simulink model "SimulinkModelGeneral_Cascaded_BAv03"  (R2022b)
settings: Solver=VariableStepAuto  StartTime=0.0  StopTime=9*3600  MaxStep=0.2  RelTol=1e-3
settings Model: NumberOfSteps=100  Creator=giaco  LastModifiedBy=giaco

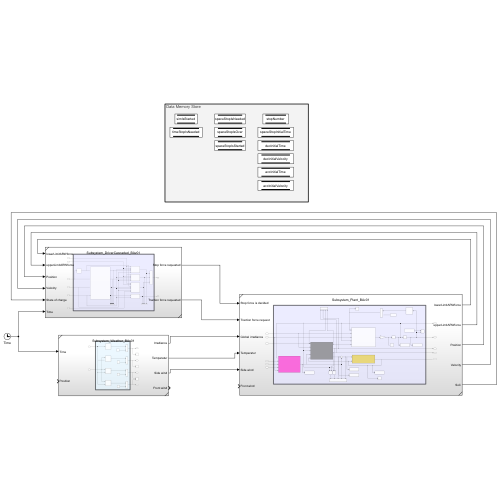
[thumbnail: Simulink's stored preview of the top-level diagram]
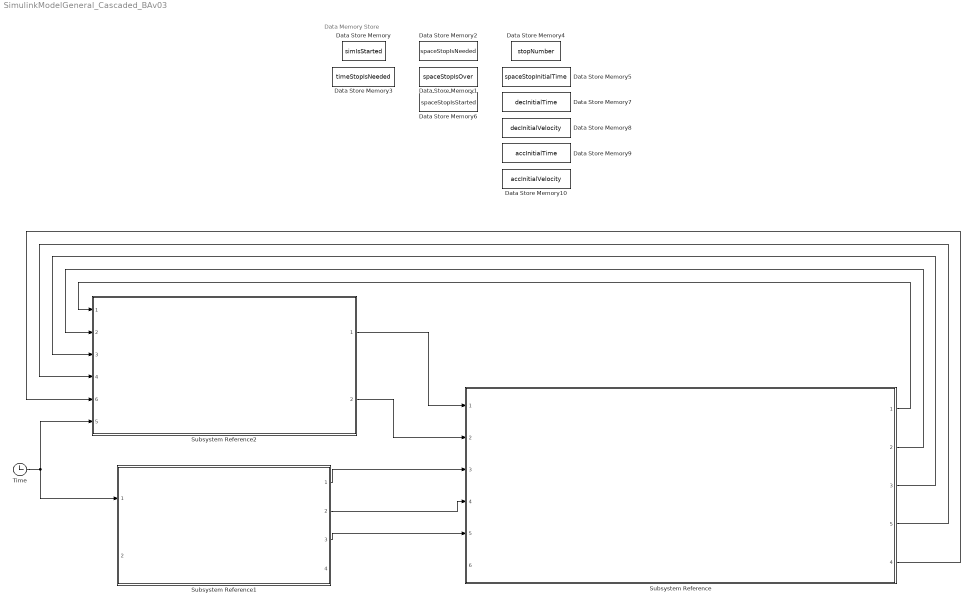
== system SimulinkModelGeneral_Cascaded_BAv03 ==
  note: Data Memory Store
  Data Store Memory : DataStoreMemory  DataStoreName=simIsStarted  WriteAfterWriteMsg=warning  InitialValue=true  ShowAdditionalParam=off  OutDataTypeStr=boolean
  Data Store Memory1 : DataStoreMemory  DataStoreName=spaceStopIsOver  WriteAfterWriteMsg=warning  InitialValue=false  ShowAdditionalParam=off  OutDataTypeStr=boolean
  Data Store Memory10 : DataStoreMemory  DataStoreName=accInitialVelocity  WriteAfterWriteMsg=warning  VectorParams1D=off  ShowAdditionalParam=off  OutDataTypeStr=double
  Data Store Memory2 : DataStoreMemory  DataStoreName=spaceStopIsNeeded  WriteAfterWriteMsg=warning  InitialValue=false  ShowAdditionalParam=off  OutDataTypeStr=boolean
  Data Store Memory3 : DataStoreMemory  DataStoreName=timeStopIsNeeded  WriteAfterWriteMsg=warning  InitialValue=false  ShowAdditionalParam=off  OutDataTypeStr=boolean
  Data Store Memory4 : DataStoreMemory  DataStoreName=stopNumber  WriteAfterWriteMsg=warning  InitialValue=2  VectorParams1D=off  ShowAdditionalParam=off  OutDataTypeStr=int8
  Data Store Memory5 : DataStoreMemory  DataStoreName=spaceStopInitialTime  WriteAfterWriteMsg=warning  VectorParams1D=off  ShowAdditionalParam=off  OutDataTypeStr=double
  Data Store Memory6 : DataStoreMemory  DataStoreName=spaceStopIsStarted  WriteAfterWriteMsg=warning  InitialValue=false  ShowAdditionalParam=off  OutDataTypeStr=boolean
  Data Store Memory7 : DataStoreMemory  DataStoreName=decInitialTime  WriteAfterWriteMsg=warning  VectorParams1D=off  ShowAdditionalParam=off  OutDataTypeStr=double
  Data Store Memory8 : DataStoreMemory  DataStoreName=decInitialVelocity  WriteAfterWriteMsg=warning  VectorParams1D=off  ShowAdditionalParam=off  OutDataTypeStr=double
  Data Store Memory9 : DataStoreMemory  DataStoreName=accInitialTime  WriteAfterWriteMsg=warning  VectorParams1D=off  ShowAdditionalParam=off  OutDataTypeStr=double
  Subsystem Reference : Subsystem  ReferencedSubsystem=Subsystem_Plant_BAv01
      settings: PortSchema="{\"entries\":[{\"content\":{\"sides\":[{\"content\":{\"connectorIds\":[\"In1\",\"In2\",\"In3\",\"In4\",\"In5\",\"In6\"]},\"type\":\"ConnectorPlacement.EquallySpacedRectSide\",\"uuid\":\"201c7402-5e26-4969-bf95-741aace5d52f\"},{\"content\":{\"connectorIds\":[\"Out1\",\"Out2\",\"Out3\",\"Out5\",\"Out4\"],\"side\":\"RIGHT\"},\"type\":\"ConnectorPlacement.EquallySpacedRectSide\",\"uuid\":\"eac15500-2534-4791-a6c9-7cdce956e4c6\"},{\"content\":{\"connectorIds\":[],\"side\":\"TOP\"},\"type\":\"ConnectorPlacement.EquallySpacedRectSide\",\"uuid\":\"55480481-707b-452f-a9f7-06d47dfb860c\"}]},\"type\":\"ConnectorPlacement.EquallySpacedConnector\",\"uuid\":\"eb257ac9-5ab4-418c-93e8-134a72900e24\"}],\"packageUris\":[\"http://schema.mathworks.com/mf0/Connector/R2020b\"],\"version\":\"1.0\"}"
  Subsystem Reference1 : Subsystem  ReferencedSubsystem=Subsystem_Weather_BAv01
  Subsystem Reference2 : Subsystem  ReferencedSubsystem=Subsystem_DriverCascaded_BAv01
      settings: PortSchema="{\"entries\":[{\"content\":{\"sides\":[{\"content\":{\"connectorIds\":[\"In1\",\"In2\",\"In3\",\"In4\",\"In6\",\"In5\"]},\"type\":\"ConnectorPlacement.EquallySpacedRectSide\",\"uuid\":\"54cb62a2-a389-4a26-af47-761a4aae3954\"},{\"content\":{\"connectorIds\":[\"Out1\",\"Out2\"],\"side\":\"RIGHT\"},\"type\":\"ConnectorPlacement.EquallySpacedRectSide\",\"uuid\":\"f9088df3-2468-42a4-b857-373d546a1026\"},{\"content\":{\"connectorIds\":[],\"side\":\"TOP\"},\"type\":\"ConnectorPlacement.EquallySpacedRectSide\",\"uuid\":\"209c9de8-7269-4c9e-a9cd-e0abbd52f09f\"}]},\"type\":\"ConnectorPlacement.EquallySpacedConnector\",\"uuid\":\"cefda859-2cec-4543-9678-4fed5dfba409\"}],\"packageUris\":[\"http://schema.mathworks.com/mf0/Connector/R2020b\"],\"version\":\"1.0\"}"
  Time : Clock
  wires:
  Subsystem Reference2/2 -> Subsystem Reference/2
  Subsystem Reference1/1 -> Subsystem Reference/3
  Subsystem Reference1/2 -> Subsystem Reference/4
  Subsystem Reference1/3 -> Subsystem Reference/5
  Time/1 -> Subsystem Reference2/5, Subsystem Reference1/1
  Subsystem Reference2/1 -> Subsystem Reference/1
  Subsystem Reference/1 -> Subsystem Reference2/1
  Subsystem Reference/2 -> Subsystem Reference2/2
  Subsystem Reference/3 -> Subsystem Reference2/3
  Subsystem Reference/5 -> Subsystem Reference2/4
  Subsystem Reference/4 -> Subsystem Reference2/6
